simulink model "project2"  (R2020a)
settings: Solver=ode45  StartTime=0.0  StopTime=10.0  RelTol=1e-3
values from neighbouring files (symbols this model uses):
  Be = 0.00612    [lab.m]    (also in prelab.m)
  compensator = (alpha*tao*s+1)/(tao*s+1)    [prelab.m]
  IntegralController = (Ki+s)/s    [lab.m]    (also in prelab.m)
  Je = 7*10^(-4)    (= 0.0007)    [lab.m]    (also in prelab.m)
  K = 12.6576    [prelab.m]
  Ka = 0.887    [lab.m]    (also in prelab.m)
  Ke = 20/(2*pi)    (= 3.18309886184)    [lab.m]    (also in prelab.m)
  Kp = 1.2527    [lab.m]    (also in prelab.m = 1/mag(W_60_index))
  Kt = 0.72    [lab.m]    (also in prelab.m)
  mu = 0.3    [lab.m]    (also in prelab.m)
  s = tf("s")    [lab.m]    (also in prelab.m)
  T = 0.0002    [lab.m]    (also in prelab.m)
libraries: cstblocks x16, simulink x2
settings Model: Creator=brucecui  LastModifiedBy=brucecui
settings SolverCC: ZeroCrossControl=DisableAll

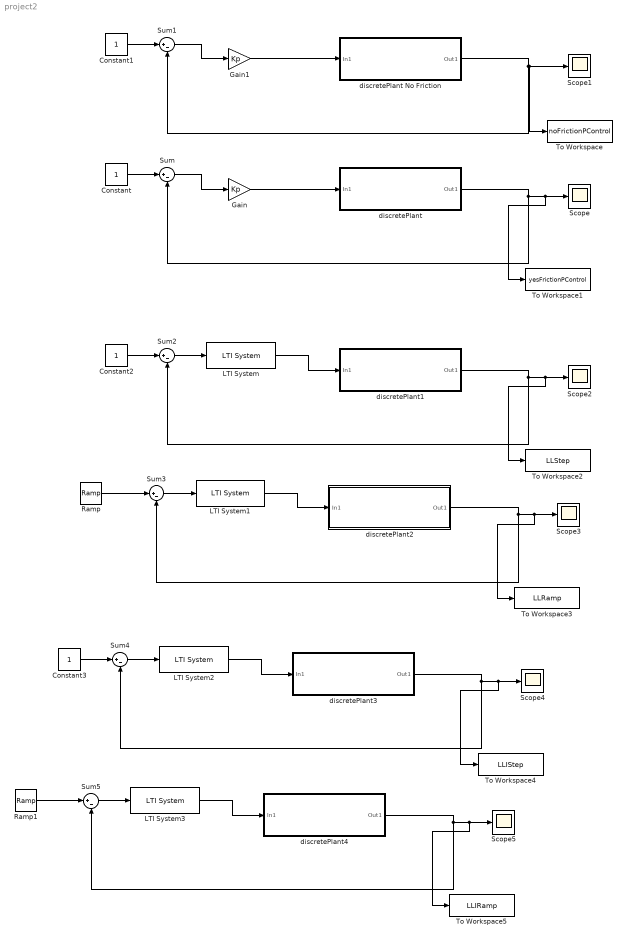
== system project2 ==
  Constant{,1..3} (4 alike) : Constant
  Gain : Gain  Gain=Kp
  Gain1 : Gain  Gain=Kp
  LTI System : cstblocks/LTI System  sys=c2d(compensator*K,T,'tustin')  IC=[]
  LTI System1 : cstblocks/LTI System  sys=c2d(compensator*K,T,'tustin')  IC=[]
  LTI System2 : cstblocks/LTI System  sys=c2d(IntegralController*compensator*K,T,'tustin')  IC=[]
  LTI System3 : cstblocks/LTI System  sys=c2d(IntegralController*compensator*K,T,'tustin')  IC=[]
  Ramp : simulink/Sources/Ramp  slope=1  start=0  InitialOutput=0
  Ramp1 : simulink/Sources/Ramp  slope=1  start=0  InitialOutput=0
  Scope{,1..5} (6 alike) : Scope
  Sum{,1..5} (6 alike) : Sum  Inputs=|+-
  To Workspace : ToWorkspace  VariableName=noFrictionPControl  SaveFormat=Timeseries  SampleTime=-1
  To Workspace1 : ToWorkspace  VariableName=yesFrictionPControl  SaveFormat=Timeseries  SampleTime=-1
  To Workspace2 : ToWorkspace  VariableName=LLStep  SaveFormat=Timeseries  SampleTime=-1
  To Workspace3 : ToWorkspace  VariableName=LLRamp  SaveFormat=Timeseries  SampleTime=-1
  To Workspace4 : ToWorkspace  VariableName=LLIStep  SaveFormat=Timeseries  SampleTime=-1
  To Workspace5 : ToWorkspace  VariableName=LLIRamp  SaveFormat=Timeseries  SampleTime=-1
  discretePlant : Subsystem
  discretePlant No Friction : Subsystem
  discretePlant1 : Subsystem
  discretePlant2 : Subsystem
  discretePlant3 : Subsystem
  discretePlant4 : Subsystem
  wires:
  Gain/1 -> discretePlant/1(In1)
  Constant/1 -> Sum/1
  Sum/1 -> Gain/1
  Gain1/1 -> discretePlant No Friction/1(In1)
  discretePlant No Friction/1(Out1) -> Scope1/1, To Workspace/1, Sum1/2
  Sum1/1 -> Gain1/1
  Constant1/1 -> Sum1/1
  discretePlant/1(Out1) -> To Workspace1/1, Scope/1, Sum/2
  LTI System/1 -> discretePlant1/1(In1)
  discretePlant1/1(Out1) -> To Workspace2/1, Scope2/1, Sum2/2
  Sum2/1 -> LTI System/1
  Constant2/1 -> Sum2/1
  discretePlant2/1(Out1) -> To Workspace3/1, Scope3/1, Sum3/2
  Sum3/1 -> LTI System1/1
  Ramp/1 -> Sum3/1
  LTI System1/1 -> discretePlant2/1(In1)
  LTI System3/1 -> discretePlant4/1(In1)
  discretePlant4/1(Out1) -> To Workspace5/1, Scope5/1, Sum5/2
  discretePlant3/1(Out1) -> To Workspace4/1, Scope4/1, Sum4/2
  Sum4/1 -> LTI System2/1
  Constant3/1 -> Sum4/1
  Sum5/1 -> LTI System3/1
  Ramp1/1 -> Sum5/1
  LTI System2/1 -> discretePlant3/1(In1)

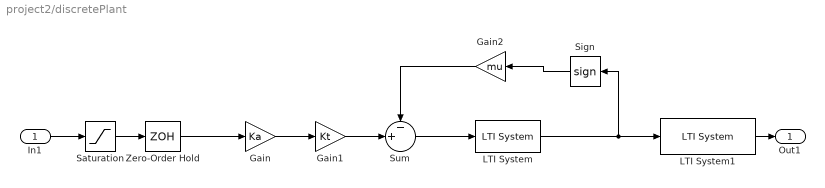
== system project2/discretePlant ==
  In1 : Inport
  Gain : Gain  Gain=Ka
  Gain1 : Gain  Gain=Kt
  Gain2 : Gain  Gain=mu
  LTI System : cstblocks/LTI System  sys=1/(Je*s+Be)  IC=[]
  LTI System1 : cstblocks/LTI System  sys=Ke/s  IC=[]
  Saturation : Saturate  UpperLimit=3  LowerLimit=-3
  Sign : Signum
  Sum : Sum  Inputs=-+|
  Zero-Order Hold : ZeroOrderHold  SampleTime=T
  Out1 : Outport
  wires:
  LTI System/1 -> LTI System1/1, Sign/1
  Zero-Order Hold/1 -> Gain/1
  Gain1/1 -> Sum/2
  Sum/1 -> LTI System/1
  Gain/1 -> Gain1/1
  Gain2/1 -> Sum/1
  Sign/1 -> Gain2/1
  LTI System1/1 -> Out1/1
  In1/1 -> Saturation/1
  Saturation/1 -> Zero-Order Hold/1

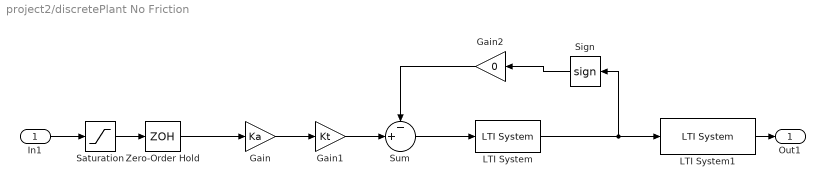
== system project2/discretePlant No Friction ==
  In1 : Inport
  Gain : Gain  Gain=Ka
  Gain1 : Gain  Gain=Kt
  Gain2 : Gain  Gain=0
  LTI System : cstblocks/LTI System  sys=1/(Je*s+Be)  IC=[]
  LTI System1 : cstblocks/LTI System  sys=Ke/s  IC=[]
  Saturation : Saturate
  Sign : Signum
  Sum : Sum  Inputs=-+|
  Zero-Order Hold : ZeroOrderHold  SampleTime=T
  Out1 : Outport
  wires:
  LTI System/1 -> LTI System1/1, Sign/1
  Zero-Order Hold/1 -> Gain/1
  Gain1/1 -> Sum/2
  Sum/1 -> LTI System/1
  Gain/1 -> Gain1/1
  Gain2/1 -> Sum/1
  Sign/1 -> Gain2/1
  LTI System1/1 -> Out1/1
  In1/1 -> Saturation/1
  Saturation/1 -> Zero-Order Hold/1

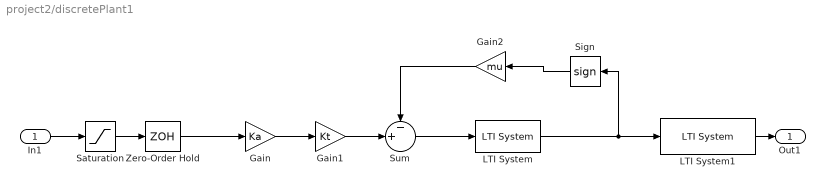
== system project2/discretePlant1 ==
  In1 : Inport
  Gain : Gain  Gain=Ka
  Gain1 : Gain  Gain=Kt
  Gain2 : Gain  Gain=mu
  LTI System : cstblocks/LTI System  sys=1/(Je*s+Be)  IC=[]
  LTI System1 : cstblocks/LTI System  sys=Ke/s  IC=[]
  Saturation : Saturate  UpperLimit=3  LowerLimit=-3
  Sign : Signum
  Sum : Sum  Inputs=-+|
  Zero-Order Hold : ZeroOrderHold  SampleTime=T
  Out1 : Outport
  wires:
  LTI System/1 -> LTI System1/1, Sign/1
  Zero-Order Hold/1 -> Gain/1
  Gain1/1 -> Sum/2
  Sum/1 -> LTI System/1
  Gain/1 -> Gain1/1
  Gain2/1 -> Sum/1
  Sign/1 -> Gain2/1
  LTI System1/1 -> Out1/1
  In1/1 -> Saturation/1
  Saturation/1 -> Zero-Order Hold/1

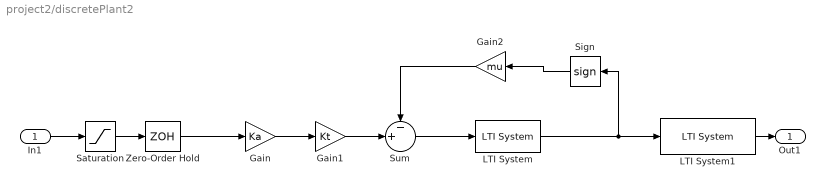
== system project2/discretePlant2 ==
  In1 : Inport
  Gain : Gain  Gain=Ka
  Gain1 : Gain  Gain=Kt
  Gain2 : Gain  Gain=mu
  LTI System : cstblocks/LTI System  sys=1/(Je*s+Be)  IC=[]
  LTI System1 : cstblocks/LTI System  sys=Ke/s  IC=[]
  Saturation : Saturate  UpperLimit=3  LowerLimit=-3
  Sign : Signum
  Sum : Sum  Inputs=-+|
  Zero-Order Hold : ZeroOrderHold  SampleTime=T
  Out1 : Outport
  wires:
  LTI System/1 -> LTI System1/1, Sign/1
  Zero-Order Hold/1 -> Gain/1
  Gain1/1 -> Sum/2
  Sum/1 -> LTI System/1
  Gain/1 -> Gain1/1
  Gain2/1 -> Sum/1
  Sign/1 -> Gain2/1
  LTI System1/1 -> Out1/1
  In1/1 -> Saturation/1
  Saturation/1 -> Zero-Order Hold/1

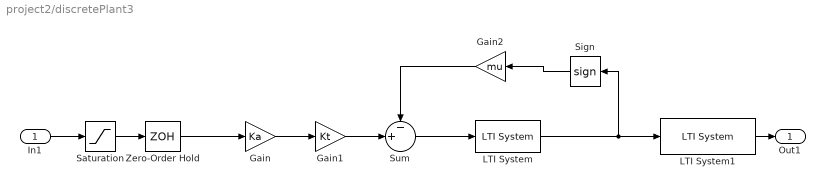
== system project2/discretePlant3 ==
  In1 : Inport
  Gain : Gain  Gain=Ka
  Gain1 : Gain  Gain=Kt
  Gain2 : Gain  Gain=mu
  LTI System : cstblocks/LTI System  sys=1/(Je*s+Be)  IC=[]
  LTI System1 : cstblocks/LTI System  sys=Ke/s  IC=[]
  Saturation : Saturate  UpperLimit=3  LowerLimit=-3
  Sign : Signum
  Sum : Sum  Inputs=-+|
  Zero-Order Hold : ZeroOrderHold  SampleTime=T
  Out1 : Outport
  wires:
  LTI System/1 -> LTI System1/1, Sign/1
  Zero-Order Hold/1 -> Gain/1
  Gain1/1 -> Sum/2
  Sum/1 -> LTI System/1
  Gain/1 -> Gain1/1
  Gain2/1 -> Sum/1
  Sign/1 -> Gain2/1
  LTI System1/1 -> Out1/1
  In1/1 -> Saturation/1
  Saturation/1 -> Zero-Order Hold/1

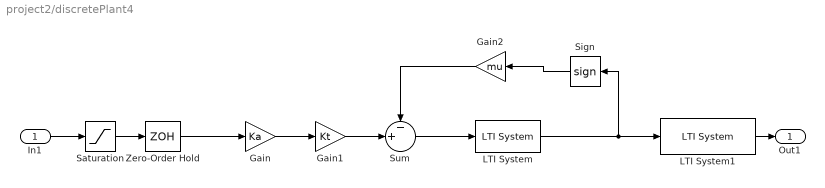
== system project2/discretePlant4 ==
  In1 : Inport
  Gain : Gain  Gain=Ka
  Gain1 : Gain  Gain=Kt
  Gain2 : Gain  Gain=mu
  LTI System : cstblocks/LTI System  sys=1/(Je*s+Be)  IC=[]
  LTI System1 : cstblocks/LTI System  sys=Ke/s  IC=[]
  Saturation : Saturate  UpperLimit=3  LowerLimit=-3
  Sign : Signum
  Sum : Sum  Inputs=-+|
  Zero-Order Hold : ZeroOrderHold  SampleTime=T
  Out1 : Outport
  wires:
  LTI System/1 -> LTI System1/1, Sign/1
  Zero-Order Hold/1 -> Gain/1
  Gain1/1 -> Sum/2
  Sum/1 -> LTI System/1
  Gain/1 -> Gain1/1
  Gain2/1 -> Sum/1
  Sign/1 -> Gain2/1
  LTI System1/1 -> Out1/1
  In1/1 -> Saturation/1
  Saturation/1 -> Zero-Order Hold/1
